simulink model "quadcopter"  (R2015b)
settings: Solver=VariableStepAuto  StartTime=0.0  StopTime=50  FixedStep=0.00001  RelTol=1e-3
libraries: simulink x4, vrlib x2
settings Model: Creator=zachn  LastModifiedBy=zachn

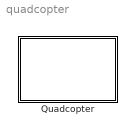
== system quadcopter ==
  Quadcopter : Subsystem  mask{m_kg=0.468, Ixyz=[4.856e-3 4.856e-3 8.801e-3], r=0.225, Kl=2.980e-6, Kb=1.140e-7, Axyz=0.25*[1 1 1], Wrpm=6100*[1 1 1 1] + 0*[-1 0 1 0] + 0*[0 -1 0 1]  + 0*[-1 1 -1 1], zdt=1, ydt_cmd=0, p_cmd=0*(pi/180), r_cmd=0*(pi/180), e0_deg=[0,0,0], e0_dot_deg=[0,0,0], x0=[0;0;0], x0_dot=[0;0;0], g=9.81}
      mask prompts: m_kg "Mass (kg)"; Ixyz "Moment of Inertia Ixyz (kg m^2)"; r "Arm Length (m)"; Kl "Lift Constant"; Kb "Rotor Drag Constant"; Axyz "Linear Aero Dynamic Drag (XYZ)"; Wrpm "Rotor Velocities (rpm)"; zdt "Z Velocity"; ydt_cmd "Yaw Rate"; p_cmd "Pitch"; r_cmd "Roll"; e0_deg "Roll, Pitch, and Yaw (deg)"; e0_dot_deg "Roll, Pitch, and Yaw Rates (deg/s)"; x0 "Position (m)"; x0_dot "Linear Velocities (m/s)"; g "Gravity Constant"
      mask init:
      | % handle mass unit conversions here
      | m = m_kg;
      | 
      | % define the inertia matrix, I, from the given components
      | I = [   Ixyz(1)     0       0   ;...
      |             0   Ixyz(2)     0   ;...
      |             0       0   Ixyz(3) ; ...
      |     ];
      | 
      | % convert open loop rotor speed inputs from rpm to radians/s
      | w_cmd = [   Wrpm(1) * (pi/30)   ; ...
      |             Wrpm(2) * (pi/30)   ; ...
      |             Wrpm(3) * (pi/30)   ; ...
      |             Wrpm(4) * (pi/30)   ; ...
      |         ];
      |     
      | % convert initial angular position and velocit from degrees to radians
      | e0 =        [   e0_deg(1)       ; ...
      |                 e0_deg(2)       ; ...
      |                 e0_deg(3)       ; ...
      |             ];
      | e0_dot =    [   e0_dot_deg(1)   ; ...
      |                 e0_dot_deg(2)   ; ...
      |                 e0_dot_deg(3)   ; ...
      |             ];
      |         
      | % create aero dynamic drag matrix
      | aero_drag = [   Axyz(1) 0   0   ; ...
      |                 0   Axyz(2) 0   ; ...
      |                 0   0   Axyz(3) ; ...
      |             ];
      mask DialogControl DescGroupVar Prompt: Quadcopter Model
      mask DialogControl Container15 Prompt: Hidden Constants

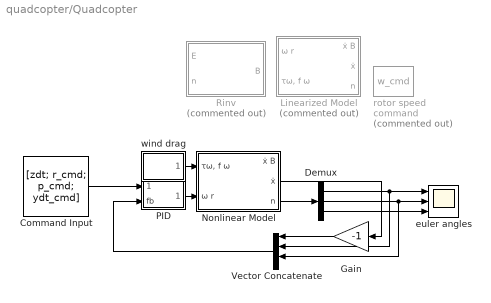
== system quadcopter/Quadcopter ==
  Command Input : Constant  Value=[zdt; r_cmd; p_cmd; ydt_cmd]  VectorParams1D=off
  Demux : Demux  Outputs=3
  Gain : Gain  Gain=-1
  Linearized Model : Subsystem  Commented=on  mask{m=m, i_xyz=Ixyz, g=g, A=0, B=0, C=0, D=0}
      mask prompts: m "Mass (kg)"; i_xyz "Moment of Inertia Ixyz (kg m^2)"; g "Gravity (m/s^2)"; A "A Matrix"; B "B Matrix"; C "C Matrix"; D "D Matrix"
      mask init:
      | A = [   zeros(3,3), eye(3,3), zeros(3,6)    ; ...
      |         zeros(3,12)                         ; ...
      |         0, -g, zeros(1,10)                  ; ...
      |         g, zeros(1,11)                      ; ...
      |         zeros(1,12)                         ; ...
      |         zeros(3,6), eye(3,3), zeros(3,3)      ...
      |     ];
      | 
      | B = [   zeros(3,4)              ; ...
      |         0, 1/i_xyz(1), 0, 0     ; ...
      |         0, 0, 1/i_xyz(2), 0     ; ...
      |         0, 0, 0, 1/i_xyz(3)     ; ...
      |         zeros(2,4)              ; ...
      |         1/m, 0, 0, 0            ; ...
      |         0,   0, 0, 0              ...
      |     ];
      | 
      | C = [   zeros(1,9),     1, zeros(1,2)   ; ...
      |         zeros(1,10),    1, zeros(1,1)   ; ...
      |         zeros(1,11),    1               ; ...
      |         zeros(1,2),     1, zeros(1,9)     ...
      |      ];
      |  
      |  D = [  zeros(3,6)                  ; ...
      |         zeros(1,3) 1/i_xyz(1) 0 0   ; ...
      |         zeros(1,4) 1/i_xyz(2) 0     ; ...
      |         zeros(1,5) 1/i_xyz(3)       ; ...
      |         1/m 0 0 0 0 0               ; ...
      |         0 1/m 0 0 0 0               ; ...
      |         0 0 1/m 0 0 0               ; ...
      |         0 0 0 1/m 0 0               ; ...
      |         zeros(3,6)                    ...
      |      ];
      mask DialogControl DescGroupVar Prompt: QUADCOPTA
      mask DialogControl DescTextVar Prompt: Linearized state space model of a four rotor quadcopter.
      mask DialogControl Control2 Prompt: GET TO THE QUADCOPTA!!!
      mask DialogControl Control2 Callback: web www.youtube.com/watch?v=Xs_OacEq2Sk
      mask DialogControl Container4 Prompt: System Parameters
  Nonlinear Model : Subsystem
  PID : Subsystem  mask{zdt_P=50, zdt_I=100, zdt_D=0, roll_P=1, roll_I=0, roll_D=0, pitch_P=1, pitch_I=0, pitch_D=0, yaw_rate_P=1, yaw_rate_I=0, yaw_rate_D=0}
      mask prompts: zdt_P "P"; zdt_I "I"; zdt_D "D"; roll_P "P"; roll_I "I"; roll_D "D"; pitch_P "P"; pitch_I "I"; pitch_D "D"; yaw_rate_P "P"; yaw_rate_I "I"; yaw_rate_D "D"
  Rinv : MATLAB Function  Commented=on  TreatAsAtomicUnit=on
  Vector Concatenate : Concatenate  NumInputs=4  Mode=Multidimensional array
  euler angles : Scope  NumInputPorts=3
  rotor speed command : Constant  Commented=on  Value=w_cmd  VectorParams1D=off
  wind drag : Subsystem
  wires:
  Demux/1 -> Vector Concatenate/2, euler angles/1
  Demux/2 -> Vector Concatenate/3, euler angles/2
  Demux/3 -> euler angles/3
  Nonlinear Model/2(ẋ) -> Gain/1
  Nonlinear Model/3(n) -> Demux/1
  Command Input/1 -> PID/1(cmd)
  Vector Concatenate/1 -> PID/2(fb)
  Gain/1 -> Vector Concatenate/1
  PID/1(ω r) -> Nonlinear Model/2(ω r)
  wind drag/1("τω, f ω ") -> Nonlinear Model/1("τω, f ω ")

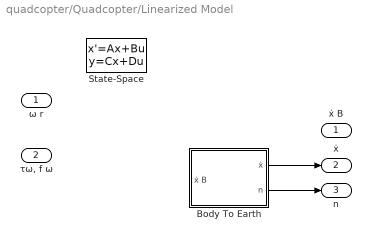
== system quadcopter/Quadcopter/Linearized Model ==
  ω r : Inport
  "τω, f ω " : Inport  Port=2
  Body To Earth : Subsystem
  State-Space : StateSpace  A=A  B=B  C=C  D=D  X0=0
  ẋ B : Outport
  ẋ : Outport  Port=2
  n : Outport  Port=3
  wires:
  Body To Earth/1(ẋ) -> ẋ/1
  Body To Earth/2(n) -> n/1

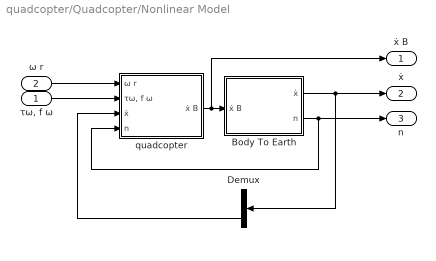
== system quadcopter/Quadcopter/Nonlinear Model ==
  "τω, f ω " : Inport
  ω r : Inport  Port=2
  Body To Earth : Subsystem
  Demux : Demux  Outputs=2
  quadcopter : Subsystem
  ẋ B : Outport
  ẋ : Outport  Port=2
  n : Outport  Port=3
  wires:
  Body To Earth/1(ẋ) -> Demux/1, ẋ/1
  ω r/1 -> quadcopter/1(ω r)
  Body To Earth/2(n) -> n/1, quadcopter/4(n)
  quadcopter/1(ẋ B) -> ẋ B/1, Body To Earth/1(ẋ B)
  "τω, f ω "/1 -> quadcopter/2("τω, f ω ")
  Demux/2 -> quadcopter/3(ẋ)

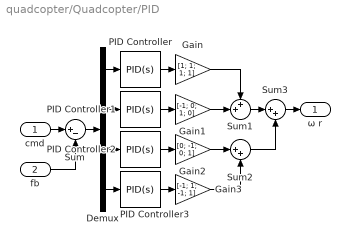
== system quadcopter/Quadcopter/PID ==
  cmd : Inport
  fb : Inport  Port=2
  Demux : Demux
  Gain : Gain  Gain=[1; 1; 1; 1]
  Gain1 : Gain  Gain=[-1; 0; 1; 0]
  Gain2 : Gain  Gain=[0; -1; 0; 1]
  Gain3 : Gain  Gain=[-1; 1; -1; 1]
  PID Controller : simulink/Continuous/PID Controller  Controller=PID  TimeDomain=Continuous-time  SampleTime=-1  IntegratorMethod=Forward Euler  FilterMethod=Forward Euler  Form=Parallel  UseFilter=on  ControllerParametersSource=internal  P=zdt_P  I=zdt_I  D=zdt_D  N=100  InitialConditionSource=internal  InitialConditionForIntegrator=0  InitialConditionForFilter=0  ExternalReset=none  LimitOutput=off  UpperSaturationLimit=inf  LowerSaturationLimit=-inf  LinearizeAsGain=on  AntiWindupMode=none  Kb=1  TrackingMode=off  Kt=1  PParamMin=[]  PParamMax=[]  IParamMin=[]  IParamMax=[]  DParamMin=[]  DParamMax=[]  NParamMin=[]  NParamMax=[]  KbParamMin=[]  KbParamMax=[]  KtParamMin=[]  KtParamMax=[]  POutMin=[]  POutMax=[]  IOutMin=[]  IOutMax=[]  DOutMin=[]  DOutMax=[]  NOutMin=[]  NOutMax=[]  KbOutMin=[]  KbOutMax=[]  KtOutMin=[]  KtOutMax=[]  IntegratorOutMin=[]  IntegratorOutMax=[]  FilterOutMin=[]  FilterOutMax=[]  SumOutMin=[]  SumOutMax=[]  SumI1OutMin=[]  SumI1OutMax=[]  SumI2OutMin=[]  SumI2OutMax=[]  SumI3OutMin=[]  SumI3OutMax=[]  SumDOutMin=[]  SumDOutMax=[]  SaturationOutMin=[]  SaturationOutMax=[]  IntegratorContinuousStateAttributes=''  IntegratorStateMustResolveToSignalObject=off  IntegratorRTWStateStorageClass=Auto  FilterContinuousStateAttributes=''  FilterStateMustResolveToSignalObject=off  FilterRTWStateStorageClass=Auto  DifferentiatorICPrevScaledInput=0  DifferentiatorOutMin=[]  DifferentiatorOutMax=[]
  PID Controller1 : simulink/Continuous/PID Controller  Controller=PID  TimeDomain=Continuous-time  SampleTime=-1  IntegratorMethod=Forward Euler  FilterMethod=Forward Euler  Form=Parallel  UseFilter=on  ControllerParametersSource=internal  P=roll_P  I=roll_I  D=roll_D  N=100  InitialConditionSource=internal  InitialConditionForIntegrator=0  InitialConditionForFilter=0  ExternalReset=none  LimitOutput=off  UpperSaturationLimit=inf  LowerSaturationLimit=-inf  LinearizeAsGain=on  AntiWindupMode=none  Kb=1  TrackingMode=off  Kt=1  PParamMin=[]  PParamMax=[]  IParamMin=[]  IParamMax=[]  DParamMin=[]  DParamMax=[]  NParamMin=[]  NParamMax=[]  KbParamMin=[]  KbParamMax=[]  KtParamMin=[]  KtParamMax=[]  POutMin=[]  POutMax=[]  IOutMin=[]  IOutMax=[]  DOutMin=[]  DOutMax=[]  NOutMin=[]  NOutMax=[]  KbOutMin=[]  KbOutMax=[]  KtOutMin=[]  KtOutMax=[]  IntegratorOutMin=[]  IntegratorOutMax=[]  FilterOutMin=[]  FilterOutMax=[]  SumOutMin=[]  SumOutMax=[]  SumI1OutMin=[]  SumI1OutMax=[]  SumI2OutMin=[]  SumI2OutMax=[]  SumI3OutMin=[]  SumI3OutMax=[]  SumDOutMin=[]  SumDOutMax=[]  SaturationOutMin=[]  SaturationOutMax=[]  IntegratorContinuousStateAttributes=''  IntegratorStateMustResolveToSignalObject=off  IntegratorRTWStateStorageClass=Auto  FilterContinuousStateAttributes=''  FilterStateMustResolveToSignalObject=off  FilterRTWStateStorageClass=Auto  DifferentiatorICPrevScaledInput=0  DifferentiatorOutMin=[]  DifferentiatorOutMax=[]
  PID Controller2 : simulink/Continuous/PID Controller  Controller=PID  TimeDomain=Continuous-time  SampleTime=-1  IntegratorMethod=Forward Euler  FilterMethod=Forward Euler  Form=Parallel  UseFilter=on  ControllerParametersSource=internal  P=pitch_P  I=pitch_I  D=pitch_D  N=100  InitialConditionSource=internal  InitialConditionForIntegrator=0  InitialConditionForFilter=0  ExternalReset=none  LimitOutput=off  UpperSaturationLimit=inf  LowerSaturationLimit=-inf  LinearizeAsGain=on  AntiWindupMode=none  Kb=1  TrackingMode=off  Kt=1  PParamMin=[]  PParamMax=[]  IParamMin=[]  IParamMax=[]  DParamMin=[]  DParamMax=[]  NParamMin=[]  NParamMax=[]  KbParamMin=[]  KbParamMax=[]  KtParamMin=[]  KtParamMax=[]  POutMin=[]  POutMax=[]  IOutMin=[]  IOutMax=[]  DOutMin=[]  DOutMax=[]  NOutMin=[]  NOutMax=[]  KbOutMin=[]  KbOutMax=[]  KtOutMin=[]  KtOutMax=[]  IntegratorOutMin=[]  IntegratorOutMax=[]  FilterOutMin=[]  FilterOutMax=[]  SumOutMin=[]  SumOutMax=[]  SumI1OutMin=[]  SumI1OutMax=[]  SumI2OutMin=[]  SumI2OutMax=[]  SumI3OutMin=[]  SumI3OutMax=[]  SumDOutMin=[]  SumDOutMax=[]  SaturationOutMin=[]  SaturationOutMax=[]  IntegratorContinuousStateAttributes=''  IntegratorStateMustResolveToSignalObject=off  IntegratorRTWStateStorageClass=Auto  FilterContinuousStateAttributes=''  FilterStateMustResolveToSignalObject=off  FilterRTWStateStorageClass=Auto  DifferentiatorICPrevScaledInput=0  DifferentiatorOutMin=[]  DifferentiatorOutMax=[]
  PID Controller3 : simulink/Continuous/PID Controller  Controller=PID  TimeDomain=Continuous-time  SampleTime=-1  IntegratorMethod=Forward Euler  FilterMethod=Forward Euler  Form=Parallel  UseFilter=on  ControllerParametersSource=internal  P=yaw_rate_P  I=yaw_rate_I  D=yaw_rate_D  N=100  InitialConditionSource=internal  InitialConditionForIntegrator=0  InitialConditionForFilter=0  ExternalReset=none  LimitOutput=off  UpperSaturationLimit=inf  LowerSaturationLimit=-inf  LinearizeAsGain=on  AntiWindupMode=none  Kb=1  TrackingMode=off  Kt=1  PParamMin=[]  PParamMax=[]  IParamMin=[]  IParamMax=[]  DParamMin=[]  DParamMax=[]  NParamMin=[]  NParamMax=[]  KbParamMin=[]  KbParamMax=[]  KtParamMin=[]  KtParamMax=[]  POutMin=[]  POutMax=[]  IOutMin=[]  IOutMax=[]  DOutMin=[]  DOutMax=[]  NOutMin=[]  NOutMax=[]  KbOutMin=[]  KbOutMax=[]  KtOutMin=[]  KtOutMax=[]  IntegratorOutMin=[]  IntegratorOutMax=[]  FilterOutMin=[]  FilterOutMax=[]  SumOutMin=[]  SumOutMax=[]  SumI1OutMin=[]  SumI1OutMax=[]  SumI2OutMin=[]  SumI2OutMax=[]  SumI3OutMin=[]  SumI3OutMax=[]  SumDOutMin=[]  SumDOutMax=[]  SaturationOutMin=[]  SaturationOutMax=[]  IntegratorContinuousStateAttributes=''  IntegratorStateMustResolveToSignalObject=off  IntegratorRTWStateStorageClass=Auto  FilterContinuousStateAttributes=''  FilterStateMustResolveToSignalObject=off  FilterRTWStateStorageClass=Auto  DifferentiatorICPrevScaledInput=0  DifferentiatorOutMin=[]  DifferentiatorOutMax=[]
  Sum : Sum  Inputs=|+-
  Sum1 : Sum  Inputs=++|
  Sum2 : Sum  Inputs=|++
  Sum3 : Sum  Inputs=|++
  ω r : Outport
  wires:
  cmd/1 -> Sum/1
  Sum/1 -> Demux/1
  Demux/2 -> PID Controller1/1
  Demux/3 -> PID Controller2/1
  Demux/4 -> PID Controller3/1
  PID Controller/1 -> Gain/1
  PID Controller1/1 -> Gain1/1
  PID Controller2/1 -> Gain2/1
  PID Controller3/1 -> Gain3/1
  Gain1/1 -> Sum1/2
  Gain/1 -> Sum1/1
  Gain2/1 -> Sum2/1
  Gain3/1 -> Sum2/2
  Sum1/1 -> Sum3/1
  Sum2/1 -> Sum3/2
  Sum3/1 -> ω r/1
  fb/1 -> Sum/2
  Demux/1 -> PID Controller/1

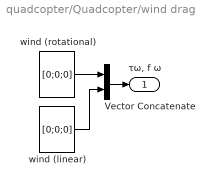
== system quadcopter/Quadcopter/wind drag ==
  Vector Concatenate : Concatenate  Mode=Multidimensional array
  wind (linear) : Constant  Value=[0;0;0]  VectorParams1D=off
  wind (rotational) : Constant  Value=[0;0;0]  VectorParams1D=off
  "τω, f ω " : Outport
  wires:
  wind (linear)/1 -> Vector Concatenate/2
  wind (rotational)/1 -> Vector Concatenate/1
  Vector Concatenate/1 -> "τω, f ω "/1

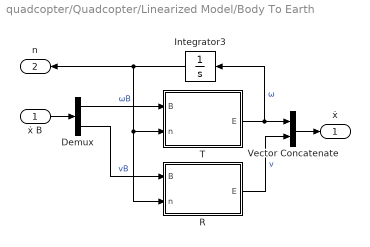
== system quadcopter/Quadcopter/Linearized Model/Body To Earth ==
  ẋ B : Inport
  Demux : Demux  Outputs=2
  Integrator3 : Integrator  InitialCondition=[0;0;0]
  R : MATLAB Function  TreatAsAtomicUnit=on
  T : MATLAB Function  TreatAsAtomicUnit=on
  Vector Concatenate : Concatenate  Mode=Multidimensional array
  ẋ : Outport
  n : Outport  Port=2
  wires:
  ẋ B/1 -> Demux/1
  Vector Concatenate/1 -> ẋ/1
  Integrator3/1 -> R/2(n), T/2(n), n/1
  T/1(E) -> Integrator3/1, Vector Concatenate/1  "ω"
  R/1(E) -> Vector Concatenate/2  "v"
  Demux/1 -> T/1(B)  "ωB"
  Demux/2 -> R/1(B)  "vB"

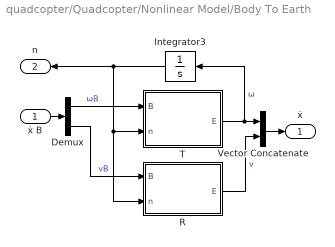
== system quadcopter/Quadcopter/Nonlinear Model/Body To Earth ==
  ẋ B : Inport
  Demux : Demux  Outputs=2
  Integrator3 : Integrator  InitialCondition=[0;0;0]
  R : MATLAB Function  TreatAsAtomicUnit=on
  T : MATLAB Function  TreatAsAtomicUnit=on
  Vector Concatenate : Concatenate  Mode=Multidimensional array
  ẋ : Outport
  n : Outport  Port=2
  wires:
  ẋ B/1 -> Demux/1
  Vector Concatenate/1 -> ẋ/1
  Integrator3/1 -> R/2(n), T/2(n), n/1
  T/1(E) -> Integrator3/1, Vector Concatenate/1  "ω"
  R/1(E) -> Vector Concatenate/2  "v"
  Demux/1 -> T/1(B)  "ωB"
  Demux/2 -> R/1(B)  "vB"

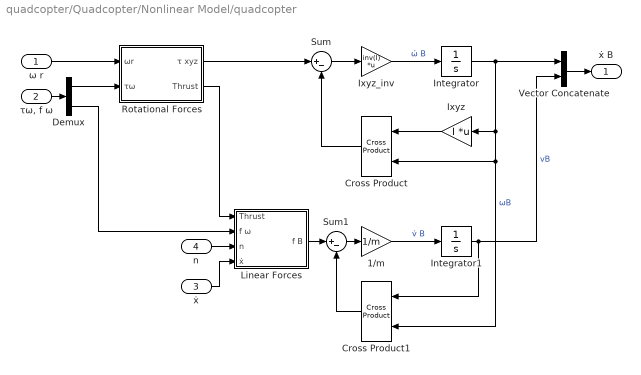
== system quadcopter/Quadcopter/Nonlinear Model/quadcopter ==
  ω r : Inport
  "τω, f ω " : Inport  Port=2
  ẋ : Inport  Port=3
  n : Inport  Port=4
  1/m : Gain  Gain=1/m
  Cross Product : vrlib/Utilities/Cross Product
  Cross Product1 : vrlib/Utilities/Cross Product
  Demux : Demux  Outputs=2
  Integrator : Integrator
  Integrator1 : Integrator
  Ixyz : Gain  Gain=I  Multiplication=Matrix(K*u)
  Ixyz_inv : Gain  Gain=inv(I)  Multiplication=Matrix(K*u)
  Linear Forces : Subsystem
  Rotational Forces : Subsystem
  Sum : Sum  Inputs=|+-
  Sum1 : Sum  Inputs=|+-
  Vector Concatenate : Concatenate  Mode=Multidimensional array
  ẋ B : Outport
  wires:
  Integrator/1 -> Cross Product1/2, Cross Product/2, Ixyz/1, Vector Concatenate/1  "ωB"
  Rotational Forces/1(τ xyz) -> Sum/1
  Integrator1/1 -> Vector Concatenate/2, Cross Product1/1  "vB"
  Sum/1 -> Ixyz_inv/1
  Ixyz_inv/1 -> Integrator/1  "ώ B"
  Ixyz/1 -> Cross Product/1
  1/m/1 -> Integrator1/1  "v̇ B"
  Cross Product/1 -> Sum/2
  Linear Forces/1(f B) -> Sum1/1
  Sum1/1 -> 1/m/1
  Cross Product1/1 -> Sum1/2
  Vector Concatenate/1 -> ẋ B/1
  n/1 -> Linear Forces/3(n)
  ω r/1 -> Rotational Forces/1(ωr)
  "τω, f ω "/1 -> Demux/1
  Demux/1 -> Rotational Forces/2(τω)
  Demux/2 -> Linear Forces/2(f ω)
  Rotational Forces/2(Thrust) -> Linear Forces/1(Thrust)
  ẋ/1 -> Linear Forces/4(ẋ)

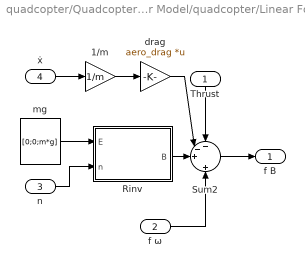
== system quadcopter/Quadcopter/Nonlinear Model/quadcopter/Linear Forces ==
  Thrust : Inport
  f ω : Inport  Port=2
  n : Inport  Port=3
  ẋ : Inport  Port=4
  1/m : Gain  Gain=1/m
  Rinv : MATLAB Function  TreatAsAtomicUnit=on
  Sum2 : Sum  Inputs=--+|+
  drag : Gain  Gain=aero_drag  Multiplication=Matrix(K*u)
  mg : Constant  Value=[0;0;m*g]  VectorParams1D=off
  f B : Outport
  wires:
  mg/1 -> Rinv/1(E)
  n/1 -> Rinv/2(n)
  f ω/1 -> Sum2/4
  Rinv/1(B) -> Sum2/3
  Sum2/1 -> f B/1
  Thrust/1 -> Sum2/1
  drag/1 -> Sum2/2
  1/m/1 -> drag/1
  ẋ/1 -> 1/m/1

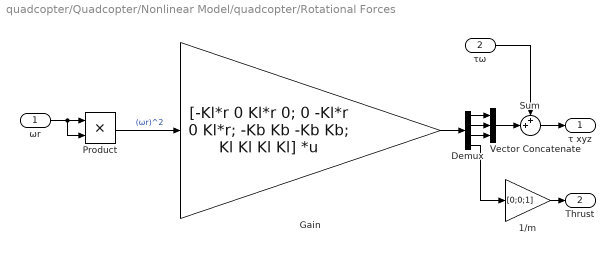
== system quadcopter/Quadcopter/Nonlinear Model/quadcopter/Rotational Forces ==
  ωr : Inport
  τω : Inport  Port=2
  1/m : Gain  Gain=[0;0;1]
  Demux : Demux
  Gain : Gain  Gain=[-Kl*r 0 Kl*r 0; 0 -Kl*r 0 Kl*r; -Kb Kb -Kb Kb; Kl Kl Kl Kl]  Multiplication=Matrix(K*u)
  Product : Product
  Sum : Sum  Inputs=++|
  Vector Concatenate : Concatenate  NumInputs=3  Mode=Multidimensional array
  τ xyz : Outport
  Thrust : Outport  Port=2
  wires:
  Demux/1 -> Vector Concatenate/1
  Demux/2 -> Vector Concatenate/2
  Demux/3 -> Vector Concatenate/3
  Gain/1 -> Demux/1
  Vector Concatenate/1 -> Sum/2
  Sum/1 -> τ xyz/1
  τω/1 -> Sum/1
  1/m/1 -> Thrust/1
  Demux/4 -> 1/m/1
  Product/1 -> Gain/1  "(ωr)^2"
  ωr/1 -> Product/2, Product/1

== matlab function quadcopter/Quadcopter/Nonlinear Model/Body To Earth/T ==
  data: B input size=[3;1]; E output; n input size=[3;1]
function E = body2euler(B,n)
% body2euler -  Given the angular velocity vector of a moving body, B,
%               returns that vector expressed in the stationary (inertial)
%               frame of reference.
%
%               'n' is the vector containing euler angles roll, pitch, and
%               yaw

phi = n(1); % roll angle
the = n(2); % pitch angle

% angular transformation matrix. This is derived using the standard yaw,
% pitch, roll seqeuence.
T = [   1   sin(phi)*tan(the)   cos(phi)*tan(the)   ; ...
        0   cos(phi)            -sin(phi)           ; ...
        0   sin(phi)/cos(the)   cos(phi)/cos(the)   ; ...
    ];

E = T * [B(1);B(2);B(3)];

== matlab function quadcopter/Quadcopter/Nonlinear Model/Body To Earth/R ==
  data: B input size=[3;1]; E output; n input size=[3;1]
function E = body2earth(B,n)
% body2earth -  translates the given vector B expressed in the moving body
%               frame to the earth (stationary or inertial) frame.
%               
%               n is the vector containing the euler angles yaw, pitch, and
%               roll.

phi = n(1); % roll (phi)
the = n(2); % pitch (theta)
psi = n(3); % yaw (psi)

c_phi = cos(phi);
s_phi = sin(phi);
c_the = cos(the);
s_the = sin(the);
c_psi = cos(psi);
s_psi = sin(psi);

% The rotation matrix using the Euler transformation ZYX
Rzyx = [
c_the*c_psi, s_phi*s_the*c_psi-c_phi*s_psi, c_phi*s_the*c_psi+s_phi*s_psi ;...
c_the*s_psi, s_phi*s_the*s_psi+c_phi*c_psi, c_phi*s_the*s_psi-s_phi*c_psi ;...
-s_the       s_phi*c_the                    c_phi*c_the                   ;...
];

E = Rzyx*[B(1);B(2);B(3)];

== matlab function quadcopter/Quadcopter/Rinv ==
  data: B output; E input; n input
function B = earth2body(E,n)
% earth2body -  Translates the given vector E expressed in the stationary
%               frame to the frame of the moving body.
%               
%               n is the vector containing the euler angles yaw, pitch, and
%               roll.

phi = n(1); % roll (phi)
the = n(2); % pitch (theta)
psi = n(3); % yaw (psi)

c_phi = cos(phi);
s_phi = sin(phi);
c_the = cos(the);
s_the = sin(the);
c_psi = cos(psi);
s_psi = sin(psi);

% The rotation matrix using the Euler transformation ZYX
Rzyx = [
c_the*c_psi, s_phi*s_the*c_psi-c_phi*s_psi, c_phi*s_the*c_psi+s_phi*s_psi ;...
c_the*s_psi, s_phi*s_the*s_psi+c_phi*c_psi, c_phi*s_the*s_psi-s_phi*c_psi ;...
-s_the       s_phi*c_the                    c_phi*c_the                   ;...
];

B = Rzyx\[E(1);E(2);E(3)];

== matlab function quadcopter/Quadcopter/Nonlinear Model/quadcopter/Linear Forces/Rinv ==
  data: B output; E input size=[3;1]; n input size=[3;1]
function B = earth2body(E,n)
% earth2body -  Translates the given vector E expressed in the stationary
%               frame to the frame of the moving body.
%               
%               n is the vector containing the euler angles yaw, pitch, and
%               roll.

phi = n(1); % roll (phi)
the = n(2); % pitch (theta)
psi = n(3); % yaw (psi)

c_phi = cos(phi);
s_phi = sin(phi);
c_the = cos(the);
s_the = sin(the);
c_psi = cos(psi);
s_psi = sin(psi);

% The rotation matrix using the Euler transformation ZYX
Rzyx = [
c_the*c_psi, s_phi*s_the*c_psi-c_phi*s_psi, c_phi*s_the*c_psi+s_phi*s_psi ;...
c_the*s_psi, s_phi*s_the*s_psi+c_phi*c_psi, c_phi*s_the*s_psi-s_phi*c_psi ;...
-s_the       s_phi*c_the                    c_phi*c_the                   ;...
];

B = Rzyx\E;

== matlab function quadcopter/Quadcopter/Linearized Model/Body To Earth/R ==
  data: B input size=[3;1]; E output; n input size=[3;1]
function E = body2earth(B,n)
% body2earth -  translates the given vector B expressed in the moving body
%               frame to the earth (stationary or inertial) frame.
%               
%               n is the vector containing the euler angles yaw, pitch, and
%               roll.

phi = n(1); % roll (phi)
the = n(2); % pitch (theta)
psi = n(3); % yaw (psi)

c_phi = cos(phi);
s_phi = sin(phi);
c_the = cos(the);
s_the = sin(the);
c_psi = cos(psi);
s_psi = sin(psi);

% The rotation matrix using the Euler transformation ZYX
Rzyx = [
c_the*c_psi, s_phi*s_the*c_psi-c_phi*s_psi, c_phi*s_the*c_psi+s_phi*s_psi ;...
c_the*s_psi, s_phi*s_the*s_psi+c_phi*c_psi, c_phi*s_the*s_psi-s_phi*c_psi ;...
-s_the       s_phi*c_the                    c_phi*c_the                   ;...
];

E = Rzyx*[B(1);B(2);B(3)];

== matlab function quadcopter/Quadcopter/Linearized Model/Body To Earth/T ==
  data: B input size=[3;1]; E output; n input size=[3;1]
function E = body2euler(B,n)
% body2euler -  Given the angular velocity vector of a moving body, B,
%               returns that vector expressed in the stationary (inertial)
%               frame of reference.
%
%               'n' is the vector containing euler angles roll, pitch, and
%               yaw

phi = n(1); % roll angle
the = n(2); % pitch angle

% angular transformation matrix. This is derived using the standard yaw,
% pitch, roll seqeuence.
T = [   1   sin(phi)*tan(the)   cos(phi)*tan(the)   ; ...
        0   cos(phi)            -sin(phi)           ; ...
        0   sin(phi)/cos(the)   cos(phi)/cos(the)   ; ...
    ];

E = T * [B(1);B(2);B(3)];
